simulink model "TP1_ROCPuente_RL"  (R2018a)
settings: Solver=ode15s  StartTime=0.0  StopTime=.1  FixedStep=1e-6  RelTol=1e-3  EnableMultiTasking=on
libraries: powerlib x15
settings Model: Creator=Monina  LastModifiedBy=Monica Romero
settings DataIOCC: LimitDataPoints=on  SaveFormat=StructureWithTime  SignalLoggingSaveFormat=ModelDataLogs  TimeSaveName=t
settings OptimizationCC: ExpressionDepthLimit=2147483647  LifeSpan=inf
settings DebuggingCC: UnderspecifiedInitializationDetection=Classic  MergeDetectMultiDrivingBlocksExec=none  SolverPrmCheckMsg=warning  FcnCallInpInsideContextMsg=warning  StateNameClashWarn=warning  SFUnexpectedBacktrackingDiag=warning  SFNoUnconditionalDefaultTransitionDiag=warning  SFExecutionAtInitializationDiag=none
settings HardwareCC: ProdBitPerPointer=32  ProdBitPerSizeT=32  ProdBitPerPtrDiffT=32  ProdLargestAtomicFloat=None  ProdIntDivRoundTo=Undefined  ProdEndianess=Unspecified  ProdWordSize=32  ProdHWDeviceType=32-bit Generic
settings ModelReferenceCC: PropagateSignalLabelsOutOfModel=off
settings CodeAppCC: StateflowObjectComments=on
settings GRTTargetCC: TargetLangStandard=C89/C90 (ANSI)  GeneratePreprocessorConditionals=Disable all  CombineOutputUpdateFcns=off  GRTInterface=on
settings ConfigComp: CovMetricSettings=dw  CovHtmlReporting=on  CovSaveCumulativeToWorkspaceVar=on  CovSaveSingleToWorkspaceVar=on  CovExternalEMLEnable=off  CovSFcnEnable=off
settings SimscapeCC: SimscapeNormalizeSystem=off

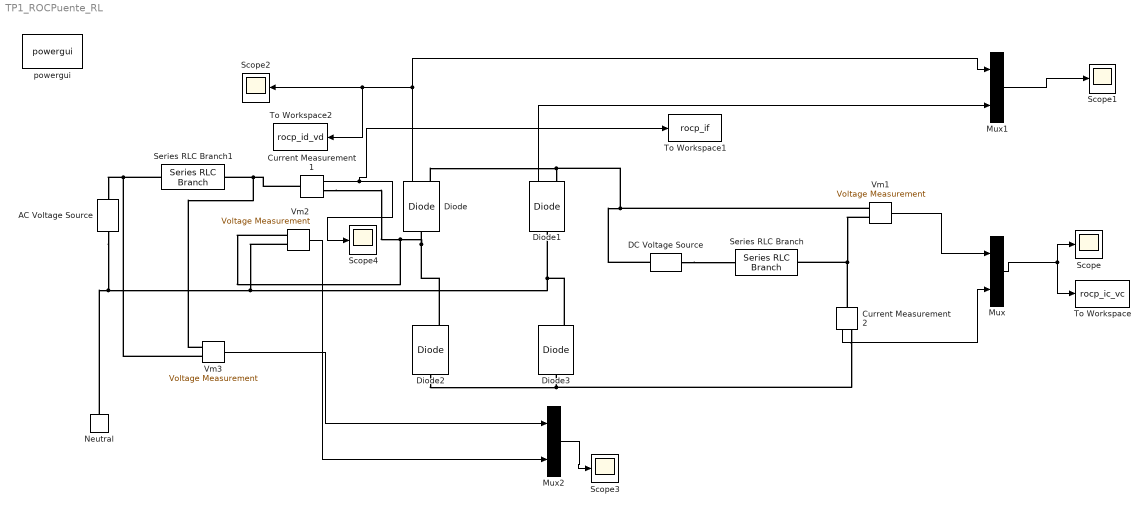
== system TP1_ROCPuente_RL ==
  AC Voltage Source : powerlib/Electrical Sources/AC Voltage Source  Amplitude=200  Phase=0  Frequency=50  SampleTime=0  Measurements=None  BusType=swing  Pref=10e3  Qref=0  Qmin=-inf  Qmax=+inf
  Current Measurement1 : powerlib/Measurements/Current Measurement  PhasorSimulation=off  OutputType=Complex  PSBequivalent=0
  Current Measurement2 : powerlib/Measurements/Current Measurement  PhasorSimulation=off  OutputType=Complex  PSBequivalent=0
  DC Voltage Source : powerlib/Electrical Sources/DC Voltage Source  Amplitude=0  Measurements=None
  Diode{,1..3} (4 alike) : powerlib/Power Electronics/Diode  Ron=0.001  Lon=0  Vf=0  IC=0  UseSnubber=off  Rs=50000  Cs=100e-12  Measurements=on
  Mux : Mux  Inputs=2
  Mux1 : Mux  Inputs=2
  Mux2 : Mux  Inputs=2
  Neutral : powerlib/Elements/Neutral  LConnTagsString=a  NodeNumber=10
      settings: SourceProductName=Simscape Power Systems  SourceProductBaseCode=PS
  Scope{,1..4} (5 alike) : Scope
  Series RLC Branch : powerlib/Elements/Series RLC Branch  LConnTagsString=__new0  RConnTagsString=__new0  BranchType=RL  Resistance=5  Inductance=.02  SetiL0=off  InitialCurrent=0  Capacitance=1.0  Setx0=off  InitialVoltage=0  Measurements=None
  Series RLC Branch1 : powerlib/Elements/Series RLC Branch  LConnTagsString=__new0  RConnTagsString=__new0  BranchType=L  Resistance=0  Inductance=.001  SetiL0=off  InitialCurrent=0  Capacitance=1.0  Setx0=off  InitialVoltage=0  Measurements=None
  To Workspace : ToWorkspace  VariableName=rocp_ic_vc  SaveFormat=Structure With Time  SampleTime=-1
  To Workspace1 : ToWorkspace  VariableName=rocp_if  SampleTime=-1
  To Workspace2 : ToWorkspace  VariableName=rocp_id_vd  SampleTime=-1
  Vm1 : powerlib/Measurements/Voltage Measurement  PhasorSimulation=off  OutputType=Complex  PSBequivalent=0
  Vm2 : powerlib/Measurements/Voltage Measurement  PhasorSimulation=off  OutputType=Complex  PSBequivalent=0
  Vm3 : powerlib/Measurements/Voltage Measurement  PhasorSimulation=off  OutputType=Complex  PSBequivalent=0
  powergui : powerlib/powergui  Priority=1  SimulationMode=Continuous  SampleTime=50e-6  frequency=60  Iterations=50  frequencyindice=50  Pbase=100e6  ErrMax=1e-4  UnitsV=kV  UnitsW=MW  buscounter=0  FunctionMessages=off  echomessages=off  EnableUseOfTLC=off  CurrentSourceSwitches=on  DisableSnubberDevices=off  DisableRonSwitches=off  DisableVfSwitches=off  DisplayEquations=off  SolverType=Tustin  Interpol=off  ExternalGateDelay=off  methode=off  Ts=0  x0status=blocks  SPID=off  SwTol=0  HookPort=off  RestoreLinks=warning  ResistiveCurrentMeasurement=off  Frange=[0:2:500]  Ylog=off  Xlog=on  ShowGrid=off  save=off  variable=ZData  structure=rocp_ic_vc  ZoomFFT=off  StartTime=0.0  cycles=1  DisplayStyle=1  fundamental=60  FreqAxis=off  MaxFrequency=1000  frequencyindicesteady=1  RmsSteady=1  display=off
  wires:
  Mux/1 -> Scope/1, To Workspace/1
  Vm1/1 -> Mux/1
  Diode/1 -> To Workspace2/1, Scope2/1, Mux1/1
  Diode1/1 -> Mux1/2
  Mux1/1 -> Scope1/1
  Current Measurement2/1 -> Mux/2
  Current Measurement1/1 -> Scope4/1, To Workspace1/1
  Mux2/1 -> Scope3/1
  Vm3/1 -> Mux2/1
  Vm2/1 -> Mux2/2
  connections:
  DC Voltage Source/LConn1 -- Series RLC Branch/RConn1
  Diode3/RConn1 -- Vm2/LConn2 -- Neutral/LConn1 -- AC Voltage Source/LConn1 -- Diode1/LConn1
  Diode/RConn1 -- DC Voltage Source/RConn1 -- Vm1/LConn1 -- Diode1/RConn1
  Diode2/LConn1 -- Current Measurement2/RConn1 -- Diode3/LConn1
  Diode2/RConn1 -- Vm2/LConn1 -- Current Measurement1/RConn1 -- Diode/LConn1
  Current Measurement2/LConn1 -- Vm1/LConn2 -- Series RLC Branch/LConn1
  Series RLC Branch1/RConn1 -- AC Voltage Source/RConn1 -- Vm3/LConn2
  Current Measurement1/LConn1 -- Vm3/LConn1 -- Series RLC Branch1/LConn1
